simulink model "beamforming"  (R2020a)
settings: Solver=VariableStepAuto  StartTime=0.0  StopTime=inf  RelTol=1e-3
values from neighbouring files (symbols this model uses):
  weights = [0.296999304879 0.3846735197 0.3846735197 0.296999304879]    [beamforming.mat]
undefined symbols (not defined in the file or in its folder): physconst
libraries: commsink2 x2, simulink x2, commdigbbndam3 x2, commchan3 x1, phaseddoalib x1, phasedtxrxlib x1, phasedbflib x1, commrandsrc3 x1, eeGeneralControl x1
settings Model: NumberOfSteps=100  Creator=jose_  LastModifiedBy=jose_

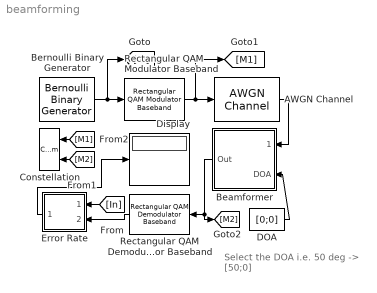
== system beamforming ==
  note: Select the DOA
      | i.e. 50 deg -> [50;0]
  AWGN Channel : commchan3/AWGN Channel  InputProcessing=Columns as channels (frame based)  seed=67  noiseMode="Signal to noise ratio  (Eb/No)"  EbNodB=30  EsNodB=10  SNRdB=10  bitsPerSym=4  Ps=1  Tsym=0.01  variance=1
  Beamformer : Subsystem
  Bernoulli Binary Generator : commrandsrc3/Bernoulli Binary Generator  ProbabilityOfZero=0.5  SeedSource=Auto  Seed=0  SampleTime=0.01/4  SamplesPerFrame=4  OutputDataType=double  SimulateUsing=Interpreted execution
  Constellation : ConstellationDiagram  NumInputPorts=2
  DOA : Constant  Value=[0;0]
  Display : Display
  Error Rate : Subsystem
  Rectangular QAM Demodulator Baseband : commdigbbndam3/Rectangular QAM Demodulator Baseband  M=16  OutType=Bit  DecType=Hard decision  VarSource=Dialog  Variance=1  Dec=Gray  Mapping=[0:15]  PowType=Min. distance between symbols  MinDist=2  AvgPow=3  PeakPow=1  Ph=0  outDtype1=Inherit via internal rule  outDtype2=Inherit via internal rule  derotateFactorWordLen=16  derotateFactorDataTypeStr=Inherit: Same word length as input  derotateFactorLastDataTypeStr=Inherit: Same word length as input  denormFactorWordLen=16  denormFactorDataTypeStr=Inherit: Same word length as input  denormFactorLastDataTypeStr=Inherit: Same word length as input  prodOutWordLen=32  prodOutOverflowMode=Wrap  prodOutRoundingMode=Floor  prodOutOvFlMode=off  prodOutOvFlModeLastStrValue=off  sumWordLen=32
  Rectangular QAM Modulator Baseband : commdigbbndam3/Rectangular QAM Modulator Baseband  M=16  InType=Bit  Enc=Gray  Mapping=[0:15]  PowType=Min. distance between symbols  MinDist=2  AvgPow=1  PeakPow=1  Ph=0  outDtype=double  outWordLen=16  outUDDataType=sfix(16)  outFracLenMode=Best precision  outFracLen=15  outDataTypeStr=double  outLastDataTypeStr=double
  wires:
  Bernoulli Binary Generator/1 -> [In], Rectangular QAM Modulator Baseband/1
  Rectangular QAM Modulator Baseband/1 -> [M1], AWGN Channel/1
  Rectangular QAM Demodulator Baseband/1 -> Error Rate/2(In2)
  Error Rate/1(Out1) -> Display/1
  [In] -> Error Rate/1(In1)
  AWGN Channel/1 -> Beamformer/1(Array Input)
  DOA/1 -> Beamformer/2(DOA)
  [M2] -> Constellation/2
  [M1] -> Constellation/1
  Beamformer/1(Out) -> Rectangular QAM Demodulator Baseband/1, [M2]

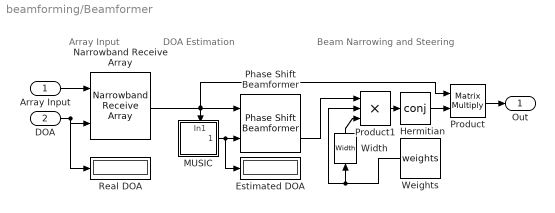
== system beamforming/Beamformer ==
  note: Beam Narrowing and Steering
  note: DOA Estimation
  note: Array Input
  Array Input : Inport
  DOA : Inport  Port=2
  Estimated DOA : Display
  Hermitian : Math  Operator=conj  SaturateOnIntegerOverflow=on
  MUSIC : Subsystem
      settings: PortSchema="{\"entries\":[{\"content\":{\"sides\":[{\"content\":{\"connectorIds\":[]},\"type\":\"ConnectorPlacement.EquallySpacedRectSide\",\"uuid\":\"2524b897-cd2a-4964-bb62-f8dc5fa407d2\"},{\"content\":{\"connectorIds\":[\"Out1\"],\"side\":\"RIGHT\"},\"type\":\"ConnectorPlacement.EquallySpacedRectSide\",\"uuid\":\"70881338-73e1-44b2-b460-f3a979bafbba\"},{\"content\":{\"connectorIds\":[\"In1\"],\"side\":\"TOP\"},\"type\":\"ConnectorPlacement.EquallySpacedRectSide\",\"uuid\":\"189e6847-bb5f-4dbc-889f-57112fcbe1ed\"}]},\"type\":\"ConnectorPlacement.EquallySpacedConnector\",\"uuid\":\"09df7b9b-c641-405d-b665-fdeae0661257\"}],\"packageUris\":[\"http://schema.mathworks.com/mf0/Connector/19700101\"],\"version\":\"1.0\"}"
  Narrowband Receive Array : phasedtxrxlib/Narrowband Receive Array  PropagationSpeed=physconst( 'LightSpeed' )  OperatingFrequency=2.4E9  Wavefront=Plane  SensorGainMeasure=dB  Polarization=None  WeightsInputPort=off  SimulateUsing=Interpreted execution  Sensor=AntennaArray
      settings: SourceProductBaseCode=AR
  Phase Shift Beamformer : phasedbflib/Phase Shift Beamformer  PropagationSpeed=physconst( 'LightSpeed' )  OperatingFrequency=2.4E9  DirectionSource=Input port  Direction=[ 0; 0 ]  NumPhaseShifterBits=0  WeightsNormalization=Distortionless  WeightsOutputPort=on  SimulateUsing=Interpreted execution  SensorArray=AntennaArray
      settings: SourceProductBaseCode=AR
  Product : Product  Multiplication=Matrix(*)
  Product1 : Product  Inputs=3
  Real DOA : Display
  Weights : Constant  Value=weights
  Width : Width
  Out : Outport
  wires:
  DOA/1 -> Real DOA/1, Narrowband Receive Array/2
  Product1/1 -> Hermitian/1
  Hermitian/1 -> Product/2
  Array Input/1 -> Narrowband Receive Array/1
  Product/1 -> Out/1
  Weights/1 -> Product1/2, Width/1
  Phase Shift Beamformer/2 -> Product1/1
  MUSIC/1(Out1) -> Estimated DOA/1, Phase Shift Beamformer/2
  Narrowband Receive Array/1 -> Product/1, MUSIC/1(In1), Phase Shift Beamformer/1
  Width/1 -> Product1/3

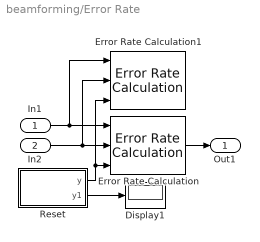
== system beamforming/Error Rate ==
  In1 : Inport
  In2 : Inport  Port=2
  Display1 : Display
  Error Rate Calculation : commsink2/Error Rate Calculation  N=0  st_delay=0  cp_mode=Entire frame  subframe=[]  PMode=Port  WsName=ErrorVec  RsMode2=on  stop=off  numErr=100  maxBits=1e6
  Error Rate Calculation1 : commsink2/Error Rate Calculation  N=0  st_delay=0  cp_mode=Entire frame  subframe=[]  PMode=Workspace  WsName=ErrorVec  RsMode2=on  stop=off  numErr=100  maxBits=1e6
  Reset : Subsystem
  Out1 : Outport
  wires:
  In1/1 -> Error Rate Calculation1/1, Error Rate Calculation/1
  Reset/1(y) -> Error Rate Calculation1/3, Error Rate Calculation/3
  Reset/2(y1) -> Display1/1
  In2/1 -> Error Rate Calculation1/2, Error Rate Calculation/2
  Error Rate Calculation/1 -> Out1/1

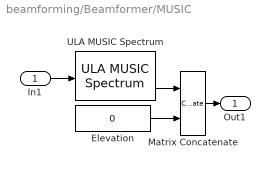
== system beamforming/Beamformer/MUSIC ==
  In1 : Inport
  Elevation : Constant  Value=0
  Matrix Concatenate : Concatenate  Mode=Multidimensional array
  ULA MUSIC Spectrum : phaseddoalib/ULA MUSIC Spectrum  PropagationSpeed=physconst( 'LightSpeed' )  OperatingFrequency=2.4E9  ForwardBackwardAveraging=off  SpatialSmoothing=0  ScanAngles=-90:90  DOAOutputPort=on  NumSignals=1  NumSignalsSource=Property  NumSignalsMethod=AIC  SimulateUsing=Interpreted execution  SensorArray=AntennaArray
      settings: SourceProductBaseCode=AR
  Out1 : Outport
  wires:
  ULA MUSIC Spectrum/2 -> Matrix Concatenate/1
  In1/1 -> ULA MUSIC Spectrum/1
  Elevation/1 -> Matrix Concatenate/2
  Matrix Concatenate/1 -> Out1/1

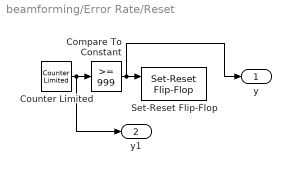
== system beamforming/Error Rate/Reset ==
  Compare To Constant : simulink/Logic and Bit Operations/Compare To Constant  relop=>=  const=999  OutDataTypeStr=boolean
  Counter Limited : simulink/Sources/Counter Limited  uplimit=1000  tsamp=1
  Set-Reset Flip-Flop : eeGeneralControl/Set-Reset Flip-Flop  LabelModeActiveChoice=Discrete  UndefState=Set  Q0=0  Ts=-1
      settings: SourceProductBaseCode=PS
  y : Outport
  y1 : Outport  Port=2
  wires:
  Counter Limited/1 -> Compare To Constant/1, y1/1
  Compare To Constant/1 -> y/1, Set-Reset Flip-Flop/1
